simulink model "quat_dyn"  (R2017b)
settings: Solver=VariableStepAuto  StartTime=0.0  StopTime=10.0  RelTol=1e-3
values from neighbouring files (symbols this model uses):
  AU = 1.496e11    (= 149600000000)    [Dyn_kin.m]    (also in trans_kin_dyn.m)
  c = SC.Polyhedron.C    [Dyn_kin.m]    (also in trans_kin_dyn.m)
  G = 6.674080000000000e-11    (= 6.67408e-11)    [Dyn_kin.m]    (also in trans_kin_dyn.m)
  mu_s = 1.326807104e20    (= 1.326807104e+20)    [Dyn_kin.m]    (also in trans_kin_dyn.m)
undefined symbols (not defined in the file or in its folder): Cube, SC, Sun
settings Model: Creator=hazr_sh  LastModifiedBy=hazr_sh

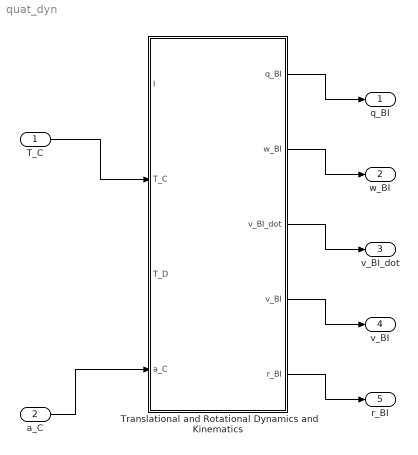
== system quat_dyn ==
  T_C : Inport
  a_C : Inport  Port=2
  Translational and Rotational Dynamics and Kinematics : Subsystem
  q_BI : Outport
  w_BI : Outport  Port=2
  v_BI_dot : Outport  Port=3
  v_BI : Outport  Port=4
  r_BI : Outport  Port=5
  wires:
  ? -> ?
  T_C/1 -> Translational and Rotational Dynamics and Kinematics/2(T_C)
  ? -> Translational and Rotational Dynamics and Kinematics/3(T_D)
  Translational and Rotational Dynamics and Kinematics/5(r_BI) -> r_BI/1
  ? -> Translational and Rotational Dynamics and Kinematics/1(I)
  Translational and Rotational Dynamics and Kinematics/4(v_BI) -> v_BI/1
  Translational and Rotational Dynamics and Kinematics/3(v_BI_dot) -> v_BI_dot/1
  a_C/1 -> Translational and Rotational Dynamics and Kinematics/4(a_C)
  Translational and Rotational Dynamics and Kinematics/2(w_BI) -> w_BI/1
  ? -> ?
  Translational and Rotational Dynamics and Kinematics/1(q_BI) -> q_BI/1
  ? -> ?

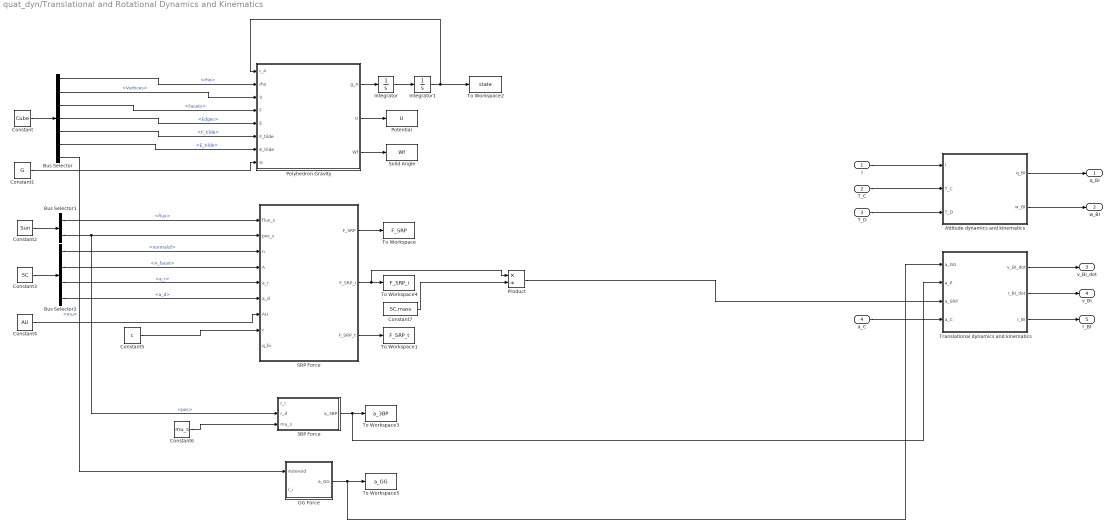
== system quat_dyn/Translational and Rotational Dynamics and Kinematics ==
  I : Inport
  T_C : Inport  Port=2
  T_D : Inport  Port=3
  a_C : Inport  Port=4
  3BP Force : MATLAB Function  TreatAsAtomicUnit=on
  Attitude dynamics and kinematics : Subsystem
  Bus Selector : BusSelector  OutputSignals=rho,Polyhedron.Vertices,Polyhedron.Facets,Polyhedron.Edges,Polyhedron.F_tilde,Polyhedron.E_tilde,mu
  Bus Selector1 : BusSelector  OutputSignals=flux,pos
  Bus Selector2 : BusSelector  OutputSignals=Polyhedron.normalsf,Polyhedron.A_facet,a_r,a_d
  Constant : Constant  Value=Cube  VectorParams1D=off  OutDataTypeStr=Bus: slBus1
  Constant1 : Constant  Value=G
  Constant2 : Constant  Value=Sun  VectorParams1D=off  OutDataTypeStr=Bus: slBus2
  Constant3 : Constant  Value=SC  VectorParams1D=off  OutDataTypeStr=Bus: slBus3
  Constant4 : Constant  Value=AU
  Constant5 : Constant  Value=c
  Constant6 : Constant  Value=mu_s
  Constant7 : Constant  Value=SC.mass
  GG Force : MATLAB Function  TreatAsAtomicUnit=on
  Integrator : Integrator  InitialCondition=SC.v_init
  Integrator1 : Integrator  InitialCondition=SC.x_init
  Polyhedron Gravity : MATLAB Function  TreatAsAtomicUnit=on
  Potential : ToWorkspace  VariableName=U  SaveFormat=Timeseries  SampleTime=-1
  Product : Product  Inputs=*/
  SRP Force : MATLAB Function  TreatAsAtomicUnit=on
  Solid Angle : ToWorkspace  VariableName=Wf  SaveFormat=Timeseries  SampleTime=-1
  To Workspace : ToWorkspace  VariableName=F_SRP  SampleTime=-1
      settings: Save2DSignal=2-D array (concatenate along first dimension)
  To Workspace1 : ToWorkspace  VariableName=F_SRP_t  SampleTime=-1
      settings: Save2DSignal=2-D array (concatenate along first dimension)
  To Workspace2 : ToWorkspace  VariableName=state  SampleTime=-1
  To Workspace3 : ToWorkspace  VariableName=a_3BP  SampleTime=-1
      settings: Save2DSignal=2-D array (concatenate along first dimension)
  To Workspace4 : ToWorkspace  VariableName=F_SRP_i  SampleTime=-1
      settings: Save2DSignal=2-D array (concatenate along first dimension)
  To Workspace5 : ToWorkspace  VariableName=a_GG  SampleTime=-1
      settings: Save2DSignal=2-D array (concatenate along first dimension)
  Translational dynamics and kinematics : Subsystem
  q_BI : Outport
  w_BI : Outport  Port=2
  v_BI_dot : Outport  Port=3
  v_BI : Outport  Port=4
  r_BI : Outport  Port=5
  wires:
  T_D/1 -> Attitude dynamics and kinematics/3(T_D)
  GG Force/1(a_GG) -> Translational dynamics and kinematics/1(a_GG), To Workspace5/1
  Product/1 -> Translational dynamics and kinematics/3(a_SRP)
  3BP Force/1(a_3BP) -> Translational dynamics and kinematics/2(a_P), To Workspace3/1
  I/1 -> Attitude dynamics and kinematics/1(I)
  Translational dynamics and kinematics/2(r_BI_dot) -> v_BI/1
  Attitude dynamics and kinematics/1(q_BI) -> q_BI/1
  T_C/1 -> Attitude dynamics and kinematics/2(T_C)
  Translational dynamics and kinematics/3(r_BI) -> r_BI/1
  Translational dynamics and kinematics/1(v_BI_dot) -> v_BI_dot/1
  Attitude dynamics and kinematics/2(w_BI) -> w_BI/1
  a_C/1 -> Translational dynamics and kinematics/4(a_C)
  Polyhedron Gravity/3(Wf) -> Solid Angle/1
  SRP Force/3(F_SRP_t) -> To Workspace1/1
  Bus Selector2/4 -> SRP Force/6(a_d)  "<a_d>"
  Bus Selector1/2 -> 3BP Force/2(r_d), SRP Force/2(pos_s)  "<pos>"
  Bus Selector/1 -> Polyhedron Gravity/2(rho)  "<rho>"
  Bus Selector/2 -> Polyhedron Gravity/3(V)  "<Vertices>"
  ? -> 3BP Force/1(r_i)
  Constant3/1 -> Bus Selector2/1
  Bus Selector2/3 -> SRP Force/5(a_r)  "<a_r>"
  Integrator1/1 -> To Workspace2/1, Polyhedron Gravity/1(r_A)
  Bus Selector/5 -> Polyhedron Gravity/6(F_tilde)  "<F_tilde>"
  Bus Selector/6 -> Polyhedron Gravity/7(E_tilde)  "<E_tilde>"
  SRP Force/2(F_SRP_i) -> Product/1, To Workspace4/1
  Constant5/1 -> SRP Force/8(c)
  Constant2/1 -> Bus Selector1/1
  Constant/1 -> Bus Selector/1
  Integrator/1 -> Integrator1/1
  Polyhedron Gravity/2(U) -> Potential/1
  Bus Selector1/1 -> SRP Force/1(flux_s)  "<flux>"
  Constant6/1 -> 3BP Force/3(mu_s)
  Bus Selector/4 -> Polyhedron Gravity/5(E)  "<Edges>"
  Constant1/1 -> Polyhedron Gravity/8(G)
  Constant4/1 -> SRP Force/7(AU)
  SRP Force/1(F_SRP) -> To Workspace/1
  Bus Selector2/2 -> SRP Force/4(A)  "<A_facet>"
  ? -> SRP Force/9(q_bi)
  Polyhedron Gravity/1(g_A) -> Integrator/1
  Bus Selector/3 -> Polyhedron Gravity/4(F)  "<Facets>"
  Bus Selector2/1 -> SRP Force/3(n)  "<normalsf>"
  Bus Selector/7 -> GG Force/1(Asteroid)  "<mu>"
  ? -> GG Force/2(r_i)
  Constant7/1 -> Product/2

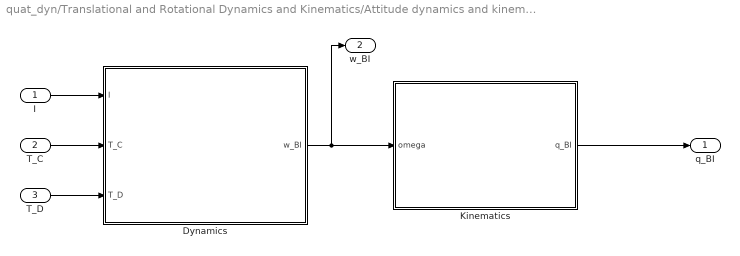
== system quat_dyn/Translational and Rotational Dynamics and Kinematics/Attitude dynamics and kinematics ==
  I : Inport
  T_C : Inport  Port=2
  T_D : Inport  Port=3
  Dynamics : Subsystem
  Kinematics : Subsystem
  q_BI : Outport
  w_BI : Outport  Port=2
  wires:
  T_C/1 -> Dynamics/2(T_C)
  Kinematics/1(q_BI) -> q_BI/1
  Dynamics/1(w_BI) -> w_BI/1, Kinematics/1(omega)
  T_D/1 -> Dynamics/3(T_D)
  I/1 -> Dynamics/1(I)

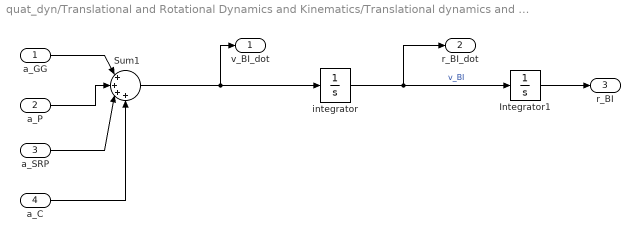
== system quat_dyn/Translational and Rotational Dynamics and Kinematics/Translational dynamics and kinematics ==
  a_GG : Inport
  a_P : Inport  Port=2
  a_SRP : Inport  Port=3
  a_C : Inport  Port=4
  " integrator" : Integrator  InitialCondition=[0,0,0]'
  Integrator1 : Integrator  InitialCondition=[0.1745 0.1745 0.1745]'
  Sum1 : Sum  Inputs=|++++
  v_BI_dot : Outport
  r_BI_dot : Outport  Port=2
  r_BI : Outport  Port=3
  wires:
  a_GG/1 -> Sum1/1
  " integrator"/1 -> r_BI_dot/1, Integrator1/1  "v_BI"
  a_P/1 -> Sum1/2
  Sum1/1 -> v_BI_dot/1, " integrator"/1
  Integrator1/1 -> r_BI/1
  a_SRP/1 -> Sum1/3
  a_C/1 -> Sum1/4

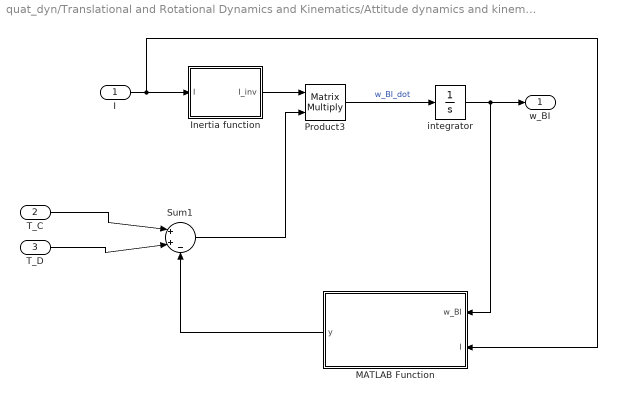
== system quat_dyn/Translational and Rotational Dynamics and Kinematics/Attitude dynamics and kinematics/Dynamics ==
  I : Inport
  T_C : Inport  Port=2
  T_D : Inport  Port=3
  " integrator" : Integrator  InitialCondition=[0,0,0]'
  "Inertia function " : MATLAB Function  TreatAsAtomicUnit=on
  MATLAB Function : MATLAB Function  TreatAsAtomicUnit=on
  Product3 : Product  Multiplication=Matrix(*)
  Sum1 : Sum  Inputs=|++-
  w_BI : Outport
  wires:
  Product3/1 -> " integrator"/1  "w_BI_dot"
  T_D/1 -> Sum1/2
  Sum1/1 -> Product3/2
  "Inertia function "/1(I_inv) -> Product3/1
  T_C/1 -> Sum1/1
  " integrator"/1 -> w_BI/1, MATLAB Function/1(w_BI)
  I/1 -> MATLAB Function/2(I), "Inertia function "/1(I)
  MATLAB Function/1(y) -> Sum1/3

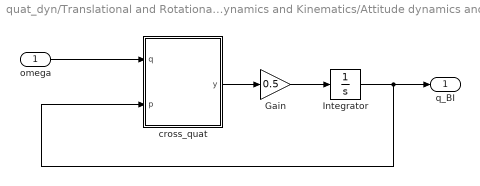
== system quat_dyn/Translational and Rotational Dynamics and Kinematics/Attitude dynamics and kinematics/Kinematics ==
  omega : Inport
  Gain : Gain  Gain=0.5
  Integrator : Integrator  InitialCondition=[0.1745 0.1745 0.1745]'
  cross_quat : MATLAB Function  TreatAsAtomicUnit=on
  q_BI : Outport
  wires:
  Integrator/1 -> cross_quat/2(p), q_BI/1
  omega/1 -> cross_quat/1(q)
  cross_quat/1(y) -> Gain/1
  Gain/1 -> Integrator/1

== matlab function quat_dyn/Translational and Rotational Dynamics and Kinematics/GG Force ==
  data: Asteroid input; a_GG output; r_i input
function a_GG = a_GG(Asteroid,r_i)

a_GG = (Asteroid.mu .* r_i)/norm(r_i)^3;

end

== matlab function quat_dyn/Translational and Rotational Dynamics and Kinematics/Attitude dynamics and kinematics/Dynamics/MATLAB Function ==
  data: w_BI input; I input; y output
function y = fcn(w_BI,I)

y = cross(w_BI, dot(I,w_BI));

end

== matlab function quat_dyn/Translational and Rotational Dynamics and Kinematics/Attitude dynamics and kinematics/Dynamics/Inertia function  ==
  data: I_inv output; I input
function I_inv = fcn(I)

I_inv = inv(I);

end

== matlab function quat_dyn/Translational and Rotational Dynamics and Kinematics/Attitude dynamics and kinematics/Kinematics/cross_quat ==
  data: q input; y output; p input
function y = cross_quat(q, p)
% Quaternion Cross Product

q4= q(4);
p4= p(4);

q_vect= q(1:3);
p_vect= p(1:3);

y = [q4.*p_vect + p4.*q_vect - cross(q_vect, p_vect); q4*p4 - dot(q_vect,p_vect)];
end

== matlab function quat_dyn/Translational and Rotational Dynamics and Kinematics/3BP Force ==
  data: r_i input; a_3BP output; r_d input; mu_s input
function a_3BP  = a_3BP(r_i,r_d,mu_s)

r_id = norm(r_d - r_i);
a_3BP = -mu_s*(r_d-r_i/r_id^3 - r_d/norm(r_d)^3); 

end

== matlab function quat_dyn/Translational and Rotational Dynamics and Kinematics/Polyhedron Gravity ==
  data: r_A input; rho input; V input; F input; E input; F_tilde input; E_tilde input; g_A output; G input; U output; Wf output
function [g_A, U, Wf] = Poly_gravity(r_A,rho,V,F,E,F_tilde,E_tilde,G)
%% Function to calculate Cube gravity from Asteroid structure (from Get_Asteroid function)
%
% Inputs: r_A - position of a field point in Asteroid frame
%         Asteroid - Asteroid structure
%
% Outputs: g_A - gravitational acceleration in Asteroid frame
%          U - gravitational potential in Asteroid frame
%          Wf - THE solid angle, which shows whether the point is in or out
%               It can be used for stopping simulation if SC crashes

%% Initialization

Wf = 0;

Facets = [0 0 0]';
Edges = [0 0 0]';

U_edg = 0;
U_fac = 0;

S = r_A;

for j=1:1:size(E,1)
    
    % Calculate gravity due to edge potential
    
    R1 = V(E(j,1),:);    
    R2 = V(E(j,2),:);    

    Ri = R1'-S;
    ri = norm(Ri);
    
    Rj = R2'-S;
    rj = norm(Rj);
        
    Rij = Rj-Ri;
    eij = norm(Rij);

    Re1 =(Ri+Rj)/2;
   
    Le = log((ri+rj+eij)/(ri+rj-eij));
    
    if Le == Inf
     
        Le = 0;
     
    end
    
    Edges = (Le*E_tilde(:,:,j)*Re1)+Edges;
    U_edg = (Le*Re1'*E_tilde(:,:,j)*Re1)+U_edg;
    
end

 for i=1:1:(size(F,1))
    
    % Calculate gravity due to face potential
    
    R1 = V(F(i,1),:);    
    R2 = V(F(i,2),:);    
    R3 = V(F(i,3),:);
    

    Ri = R1'-S;
    ri = norm(Ri);
    
    Rj = R2'-S;
    rj = norm(Rj);
    
    Rk = R3'-S;
    rk = norm(Rk);
    
    
    wf = 2*atan2(dot(Ri, cross(Rj,Rk)),(ri*rj*rk+ri*dot(Rj,Rk)+rj*dot(Rk,Ri)+rk*dot(Ri,Rj)));
    
    Rf =(Ri+Rj+Rk)/3;

    U_fac = wf*Rf'*F_tilde(:,:,i)*Rf+U_fac;
    Facets = wf*F_tilde(:,:,i)*Rf+Facets;
    
    Wf = wf+Wf;
  
 end

g_A = G*rho*(-Edges+Facets);

U = 0.5*G*rho*(U_edg-U_fac);

end

== matlab function quat_dyn/Translational and Rotational Dynamics and Kinematics/SRP Force ==
  data: flux_s input; pos_s input; n input; A input; a_r input; a_d input; AU input; c input; F_SRP output; F_SRP_i output; F_SRP_t output; q_bi input
function [F_SRP,F_SRP_i,F_SRP_t]   = F_SRP(flux_s,pos_s,n,A,a_r,a_d,AU,c,q_bi)

e = pos_s(1,1:3)/norm(pos_s(1,1:3));
P = flux_s/(norm(pos_s(1,1:3)/AU)^2*c);

F_SRP = zeros(size(n,1),3); 
for i=1:1:size(n,1)
    
    co = dot(n(i,1:3),e(1,1:3),2);

    if i<=12
        F = -P*A(i,:)*co.*((2*(a_d(1,1)/3 + a_r(1,1)*co))'.*n(i,1:3) + (1-a_r(1,1))'.*e);
        F_SRP(i,:) = F;
    else
        F = -P*A(i,:)*co.*((2*(a_d(1,2)/3 + a_r(1,2)*co))'.*n(i,1:3) + (1-a_r(1,2))'.*e);
        F_SRP(i,:) = F;
    end
    
    
end
% 
F_SRP_i = cross_quat(q_bi,cross_quat([F_SRP 0]',conj_quat(q_bi)));
F_SRP_t = sum(F_SRP);

end
